simulink model "merge_test_tmp"  (Simulink 8.5)
settings: Solver=VariableStepDiscrete  StartTime=0.0  StopTime=20  MaxStep=1  RelTol=1e-3
settings Model: Creator=arnaud  LastModifiedBy=hbourbou  CovSFcnEnable=off
settings DataIOCC: ExternalInput=xin  SaveFormat=Structure
settings DebuggingCC: SolverPrmCheckMsg=warning  FcnCallInpInsideContextMsg=EnableAllAsWarning

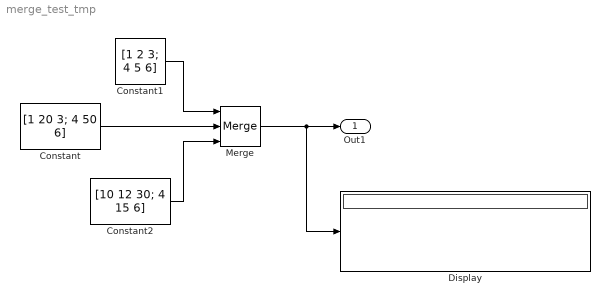
== system merge_test_tmp ==
  Constant : Constant  Value=[1 20 3; 4 50 6]
  Constant1 : Constant  Value=[1 2 3; 4 5 6]
  Constant2 : Constant  Value=[10 12 30; 4 15 6]
  Display : Display
  Merge : Merge  Inputs=3
  Out1 : Outport
  wires:
  Merge/1 -> Display/1, Out1/1
  Constant1/1 -> Merge/1
  Constant/1 -> Merge/2
  Constant2/1 -> Merge/3
